simulink model "VSI_C_Simulation_Blocks"  (R2025b)
settings: Solver=VariableStepAuto  StartTime=0.0  StopTime=0.3  FixedStep=Ts  RelTol=1e-3
values from neighbouring files (symbols this model uses):
  A = [-Rf/Lf  w     -1/Lf   0 ... (first row only)    [VSI_C_Init.m]
  B = [1/Lf   0 ... (first row only)    [VSI_C_Init.m]
  C = eye(nx)    [VSI_C_Init.m]
  Hx = [0 0 1 0 ... (first row only)    [VSI_C_Init.m]
  K = dlqr(Ad_aug,Bd_aug,Q,R)    [VSI_C_Init.m]
  nu = size(B,2)    [VSI_C_Init.m]
  nx = size(B,1)    [VSI_C_Init.m]
  P = [ 0     0 ... (first row only)    [VSI_C_Init.m]
  Ts = 1/fsw    (= 0.0002)    [VSI_C_Init.m]
undefined symbols (not defined in the file or in its folder): DiscIntNeverNeededParam, plecs
settings Model: Creator=dfigueroa  LastModifiedBy=dfigueroa

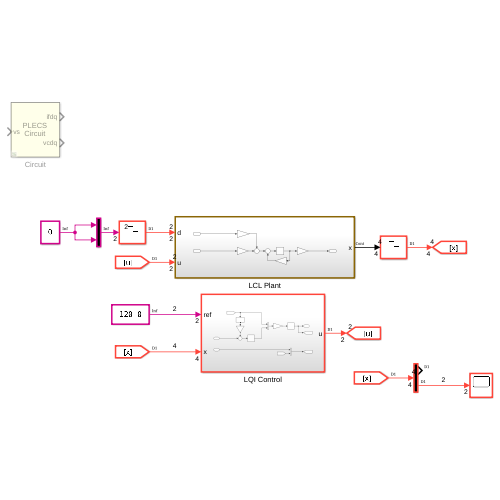
[thumbnail: Simulink's stored preview of the top-level diagram]
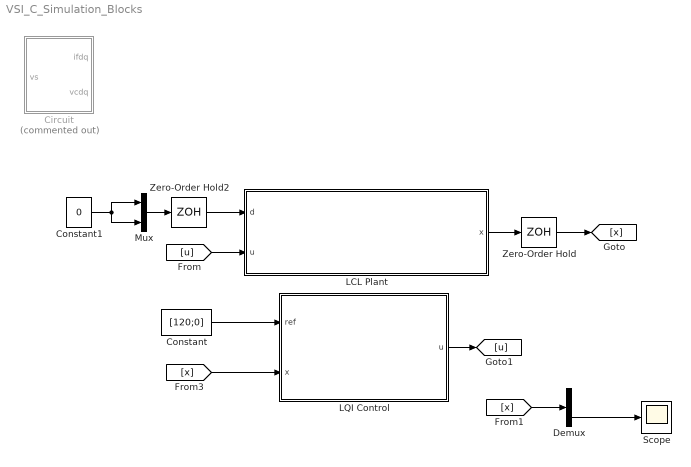
== system VSI_C_Simulation_Blocks ==
  Circuit : Subsystem  Commented=on  LoadFcn=plecs('sl', 200);  InitFcn=plecs('sl', 214);  StartFcn=plecs('sl', 208);  StopFcn=plecs('sl', 209);  ClipboardFcn=plecs('sl', 212, 4);  mask(PlecsCircuit){PLECSData=<binary blob, 2876 chars, not shown>}
      mask prompts: PLECSData "PLECS Data (Do not delete or modify!)"
      mask init:
      | % PLACE CUSTOM INITIALIZATIONS ABOVE
      | % DO NOT REMOVE
      | plecs('sl', 215);
      | % DO NOT REMOVE
      settings: CopyFcn=plecs('sl', 203);  DeleteFcn=plecs('sl', 205);  UndoDeleteFcn=plecs('sl', 206);  PreSaveFcn=plecs('sl', 211);  PostSaveFcn=plecs('sl', 201);  NameChangeFcn=plecs('sl', 210);  DestroyFcn=plecs('sl', 207);  PreCopyFcn=plecs('sl', 216);  OpenFcn=plecs('sl', 202);  ErrorFcn=plerrorfcn
      mask Help: eval('plecs(''help'', ''qthelp:///creatingacircuit.html'')')
      mask Display: disp('PLECS\nCircuit')
  Constant : Constant  Value=[120;0]
  Constant1 : Constant  Value=0
  Demux : Demux  Outputs=2
  LCL Plant : Subsystem
  LQI Control : Subsystem
  Mux : Mux  Inputs=2
  Scope : Scope
      settings: ActiveDisplayYMinimum=-15.240269745984477  ActiveDisplayYMaximum=135.02669588680592
  Zero-Order Hold : ZeroOrderHold  SampleTime=Ts
  Zero-Order Hold2 : ZeroOrderHold  SampleTime=Ts
  wires:
  Demux/2 -> Scope/1
  [x] -> Demux/1
  Zero-Order Hold/1 -> [x]
  Zero-Order Hold2/1 -> LCL Plant/1(d)
  LCL Plant/1(x) -> Zero-Order Hold/1
  [u] -> LCL Plant/2(u)
  Constant/1 -> LQI Control/1(ref)
  [x] -> LQI Control/2(x)
  LQI Control/1(u) -> [u]
  Mux/1 -> Zero-Order Hold2/1
  Constant1/1 -> Mux/1, Mux/2

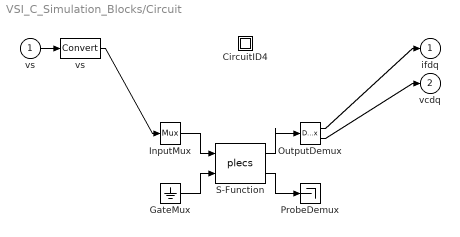
== system VSI_C_Simulation_Blocks/Circuit ==
  vs : Inport  PortDimensions=2
  " CircuitID4 " : Subsystem
  " GateMux " : Ground
  " InputMux " : Mux  Inputs=[ 2 ]
  " OutputDemux " : Demux  Outputs=[ 2 2 ]
  " ProbeDemux " : Terminator
  " S-Function " : S-Function  FunctionName=plecs  SFunctionDeploymentMode=off  EnableBusSupport=off
  " vs " : DataTypeConversion
  ifdq : Outport  PortDimensions=2
  vcdq : Outport  Port=2  PortDimensions=2
  wires:
  " S-Function "/1 -> " OutputDemux "/1
  " InputMux "/1 -> " S-Function "/1
  " GateMux "/1 -> " S-Function "/2
  " S-Function "/2 -> " ProbeDemux "/1
  vs/1 -> " vs "/1
  " vs "/1 -> " InputMux "/1
  " OutputDemux "/1 -> ifdq/1
  " OutputDemux "/2 -> vcdq/1

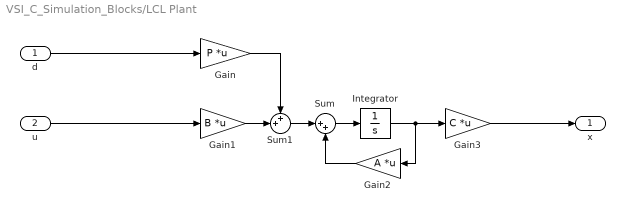
== system VSI_C_Simulation_Blocks/LCL Plant ==
  d : Inport
  u : Inport  Port=2
  Gain : Gain  Gain=P  Multiplication=Matrix(K*u)
  Gain1 : Gain  Gain=B  Multiplication=Matrix(K*u)
  Gain2 : Gain  Gain=A  Multiplication=Matrix(K*u)
  Gain3 : Gain  Gain=C  Multiplication=Matrix(K*u)
  Integrator : Integrator
  Sum : Sum  Inputs=|++
  Sum1 : Sum  Inputs=++|
  x : Outport
  wires:
  u/1 -> Gain1/1
  Gain2/1 -> Sum/2
  Gain/1 -> Sum1/1
  Sum/1 -> Integrator/1
  Integrator/1 -> Gain3/1, Gain2/1
  d/1 -> Gain/1
  Sum1/1 -> Sum/1
  Gain1/1 -> Sum1/2
  Gain3/1 -> x/1

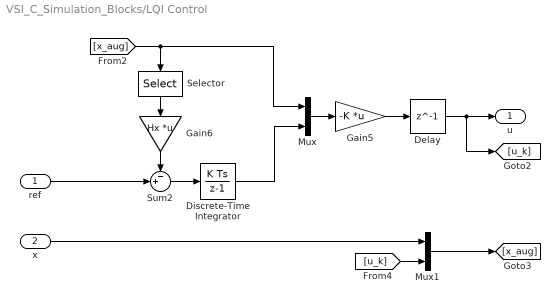
== system VSI_C_Simulation_Blocks/LQI Control ==
  ref : Inport
  x : Inport  Port=2
  Delay : Delay  DelayLength=1  SampleTime=Ts
  Discrete-Time Integrator : DiscreteIntegrator  SampleTime=Ts  ICPrevOutput=DiscIntNeverNeededParam  ICPrevScaledInput=DiscIntNeverNeededParam
  Gain5 : Gain  Gain=-K  Multiplication=Matrix(K*u)
  Gain6 : Gain  Gain=Hx  Multiplication=Matrix(K*u)
  Mux : Mux  Inputs=[(nx + nu) 2]
  Mux1 : Mux  Inputs=[nx nu]
  Selector : Selector  InputPortWidth=6  IndexOptions=Index vector (dialog)  Indices=[1 2 3 4]  OutputSizes=1
  Sum2 : Sum  Inputs=-+|
  u : Outport
  wires:
  Mux/1 -> Gain5/1
  Discrete-Time Integrator/1 -> Mux/2
  Gain5/1 -> Delay/1
  [u_k] -> Mux1/2
  Mux1/1 -> [x_aug]
  Selector/1 -> Gain6/1
  Gain6/1 -> Sum2/1
  Sum2/1 -> Discrete-Time Integrator/1
  Delay/1 -> u/1, [u_k]
  x/1 -> Mux1/1
  [x_aug] -> Mux/1, Selector/1
  ref/1 -> Sum2/2

== system VSI_C_Simulation_Blocks/Circuit/ CircuitID4  ==
